simulink model "SimilinkPIDModel"  (R2017b)
settings: Solver=VariableStepAuto  StartTime=0.0  StopTime=250  RelTol=1e-3
settings Model: Creator=olavoie  LastModifiedBy=olavoie

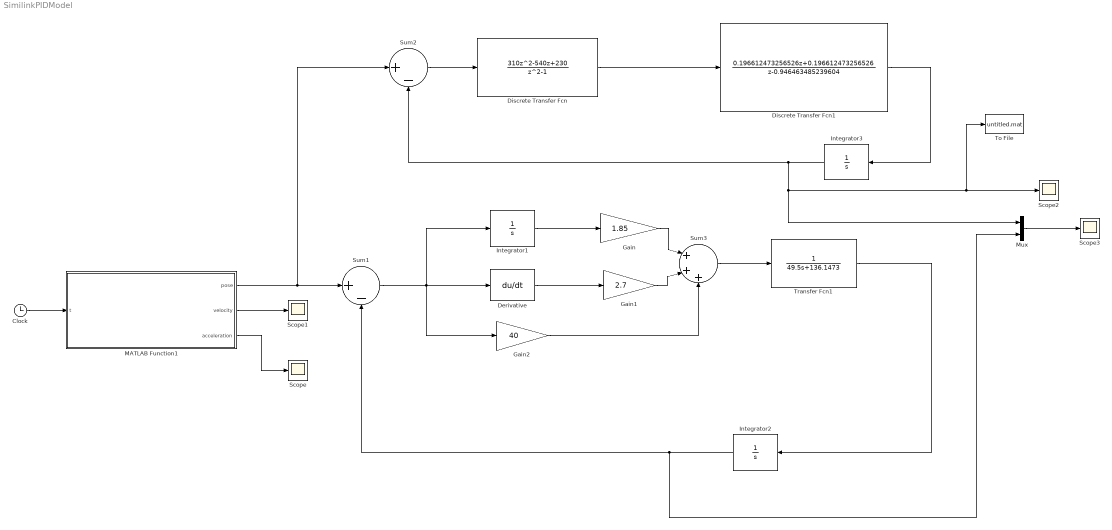
== system SimilinkPIDModel ==
  Clock : Clock
      settings: Decimation=2
  Derivative : Derivative
  Discrete Transfer Fcn : DiscreteTransferFcn  Numerator=[310 -540 230]  Denominator=[1 0 -1]  SampleTime=0.02
  Discrete Transfer Fcn1 : DiscreteTransferFcn  Numerator=[0.196612473256526 0.196612473256526]  Denominator=[1 -0.946463485239604]  SampleTime=0.02
  Gain : Gain  Gain=1.85
  Gain1 : Gain  Gain=2.7
  Gain2 : Gain  Gain=40
  Integrator1 : Integrator
  Integrator2 : Integrator
  Integrator3 : Integrator
  MATLAB Function1 : MATLAB Function  TreatAsAtomicUnit=on
  Mux : Mux  Inputs=2
  Scope{,1..3} (4 alike) : Scope
  Sum1 : Sum  Inputs=|+-
  Sum2 : Sum  Inputs=|+-
  Sum3 : Sum  Inputs=|+++
  To File : ToFile
      settings: Decimation=20
  Transfer Fcn1 : TransferFcn  Denominator=[49.5 136.1473]
  wires:
  Gain/1 -> Sum3/1
  Gain2/1 -> Sum3/3
  Integrator1/1 -> Gain/1
  Derivative/1 -> Gain1/1
  Gain1/1 -> Sum3/2
  Clock/1 -> MATLAB Function1/1(t)
  MATLAB Function1/1(pose) -> Sum2/1, Sum1/1
  Integrator2/1 -> Mux/2, Sum1/2
  MATLAB Function1/2(velocity) -> Scope1/1
  MATLAB Function1/3(acceleration) -> Scope/1
  Discrete Transfer Fcn/1 -> Discrete Transfer Fcn1/1
  Sum3/1 -> Transfer Fcn1/1
  Sum1/1 -> Gain2/1, Derivative/1, Integrator1/1
  Transfer Fcn1/1 -> Integrator2/1
  Sum2/1 -> Discrete Transfer Fcn/1
  Discrete Transfer Fcn1/1 -> Integrator3/1
  Integrator3/1 -> To File/1, Scope2/1, Mux/1, Sum2/2
  Mux/1 -> Scope3/1

== matlab function SimilinkPIDModel/MATLAB Function1 ==
  data: pose output; velocity output; acceleration output; t input

function [pose, velocity, acceleration] = SimulinkTrajectoryGenerator(t)
    timeStamp      = 0.02;
    TrajectoryTime = 3;
    startPose      = 0;
    endPose        = 2;

    j = t * timeStamp;
    if j > TrajectoryTime
        j = TrajectoryTime;
    end
    pose         = poseTrajectory(j, startPose, endPose, TrajectoryTime);
    velocity     = velocityTrajectory(j, startPose, endPose, TrajectoryTime);
    acceleration = accelarationTrajectory(j, startPose, endPose, TrajectoryTime);
    
    if j >= TrajectoryTime
        acceleration = 0.0;
    end
    
end


function y = poseTrajectory(t, P0, P1, timeResponse)
    spline_time_squared = t^2;
    spline_time_cubed   = t^3;
    t_f_squared = timeResponse^2;
    t_f_cubed   = timeResponse^3;
    
    y = P0 + (3 / t_f_squared) * (P1 - P0) * spline_time_squared + (-2 / t_f_cubed) * (P1 - P0) * spline_time_cubed;

end

function y = velocityTrajectory(t, P0, P1, timeResponse)
    spline_time         = t;
    spline_time_squared = t^2;
    t_f_squared = timeResponse^2;
    t_f_cubed   = timeResponse^3;
    
    y = 2 * (3 / t_f_squared) * (P1 - P0) * spline_time + 3 * (-2 / t_f_cubed) * (P1 - P0) * spline_time_squared;

end

function y = accelarationTrajectory(t, P0, P1, timeResponse)
    spline_time         = t;
    t_f_squared = timeResponse^2;
    t_f_cubed   = timeResponse^3;
    
    y = 2 * (3 / t_f_squared) * (P1 - P0) + 6 * (-2 / t_f_cubed) * (P1 - P0) * spline_time;
end
